simulink model "windturbinemod"  (Simulink 10.0)
settings: Solver=ode45  StartTime=0.0  StopTime=150  RelTol=1e-3  EnableMultiTasking=on
libraries: simulink x1
settings Model: Creator=dinu  LastModifiedBy=bhisma
settings DataIOCC: LimitDataPoints=on  SignalLoggingSaveFormat=ModelDataLogs
settings OptimizationCC: ExpressionDepthLimit=2147483647  InitFltsAndDblsToZero=on
settings DebuggingCC: SaveWithParameterizedLinksMsg=none  SignalResolutionControl=TryResolveAllWithWarning  SolverPrmCheckMsg=warning  MultiTaskDSMMsg=warning  MultiTaskCondExecSysMsg=none  FcnCallInpInsideContextMsg=warning  StateNameClashWarn=warning
settings GRTTargetCC: TargetFcnLib=ansi_tfl_tmw.mat  GeneratePreprocessorConditionals=Disable all
settings ConfigComp: CovExternalEMLEnable=off

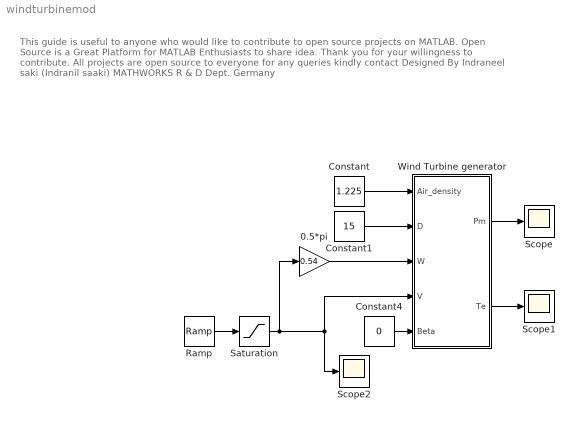
== system windturbinemod ==
  note: This guide is useful to anyone who would like to contribute to open source projects on MATLAB.
      | Open Source is a Great Platform for MATLAB Enthusiasts to share idea. Thank you for your willingness to contribute.
      | All projects are open source to everyone for any queries kindly contact
      | Designed By Indraneel saki (Indranil saaki)
      | MATHWORKS R & D Dept.
      | Germany
  0.5*pi : Gain  Gain=0.54
  Constant : Constant  Value=1.225
  Constant1 : Constant  Value=15
  Constant4 : Constant  Value=0
  Ramp : simulink/Sources/Ramp  SystemSampleTime=-1  slope=1  start=0  X0=0
  Saturation : Saturate  UpperLimit=100  LowerLimit=3
  Scope : Scope
  Scope1 : Scope
  Scope2 : Scope
  Wind Turbine generator : Subsystem
  wires:
  Wind Turbine generator/1(Pm) -> Scope/1
  Constant/1 -> Wind Turbine generator/1(Air_density)
  Constant1/1 -> Wind Turbine generator/2(D)
  Saturation/1 -> 0.5*pi/1, Wind Turbine generator/4(V), Scope2/1
  Constant4/1 -> Wind Turbine generator/5(Beta)
  Wind Turbine generator/2(Te) -> Scope1/1
  Ramp/1 -> Saturation/1
  0.5*pi/1 -> Wind Turbine generator/3(W)

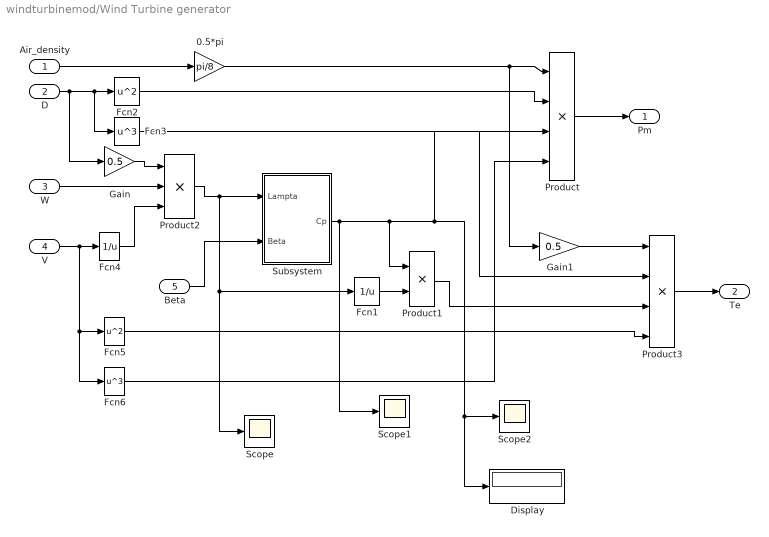
== system windturbinemod/Wind Turbine generator ==
  Air_density : Inport
  D : Inport  Port=2
  W : Inport  Port=3
  V : Inport  Port=4
  Beta : Inport  Port=5
  0.5*pi : Gain  Gain=pi/8
  Display : Display
  Fcn1 : Fcn  Expr=1/u
  Fcn2 : Fcn  Expr=u^2
  Fcn3 : Fcn  Expr=u^3
  Fcn4 : Fcn  Expr=1/u
  Fcn5 : Fcn  Expr=u^2
  Fcn6 : Fcn  Expr=u^3
  Gain : Gain  Gain=0.5
  Gain1 : Gain  Gain=0.5
  Product : Product  Inputs=4  RndMeth=Zero
  Product1 : Product  RndMeth=Zero
  Product2 : Product  Inputs=3  RndMeth=Zero
  Product3 : Product  Inputs=4  RndMeth=Zero
  Scope : Scope
  Scope1 : Scope
  Scope2 : Scope
  Subsystem : Subsystem
  Pm : Outport
  Te : Outport  Port=2
  wires:
  Air_density/1 -> 0.5*pi/1
  D/1 -> Fcn2/1, Fcn3/1, Gain/1
  W/1 -> Product2/2
  V/1 -> Fcn4/1, Fcn5/1, Fcn6/1
  Fcn4/1 -> Product2/3
  Product/1 -> Pm/1
  Fcn2/1 -> Product/2
  Beta/1 -> Subsystem/2(Beta)
  Product2/1 -> Subsystem/1(Lampta), Fcn1/1, Scope/1
  Subsystem/1(Cp) -> Product1/1, Product/3, Scope2/1, Display/1, Scope1/1
  Fcn1/1 -> Product1/2
  Product1/1 -> Product3/3
  Fcn3/1 -> Product3/2
  Fcn5/1 -> Product3/4
  Fcn6/1 -> Product/4
  Product3/1 -> Te/1
  0.5*pi/1 -> Product/1, Gain1/1
  Gain/1 -> Product2/1
  Gain1/1 -> Product3/1

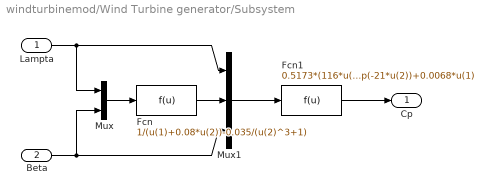
== system windturbinemod/Wind Turbine generator/Subsystem ==
  Lampta : Inport
  Beta : Inport  Port=2
  Fcn : Fcn  Expr=1/(u(1)+0.08*u(2))-0.035/(u(2)^3+1)
  Fcn1 : Fcn  Expr=0.5173*(116*u(2)-0.4*u(3)-5)*exp(-21*u(2))+0.0068*u(1)
  Mux : Mux  Inputs=2
  Mux1 : Mux  Inputs=3
  Cp : Outport
  wires:
  Mux/1 -> Fcn/1
  Fcn/1 -> Mux1/2
  Mux1/1 -> Fcn1/1
  Fcn1/1 -> Cp/1
  Beta/1 -> Mux/2, Mux1/3
  Lampta/1 -> Mux/1, Mux1/1
